simulink model "serial_send"  (R2018a)
settings: Solver=FixedStepAuto  StartTime=0.0  StopTime=1000000  FixedStep=0.01  RelTol=1e-3
undefined symbols (not defined in the file): serial
libraries: instrumentlib x2
settings Model: Creator=SIMONE  LastModifiedBy=SIMONE

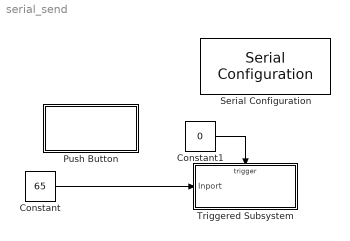
== system serial_send ==
  Constant : Constant  Value=65  OutDataTypeStr=uint8
  Constant1 : Constant  Value=0
  Push Button : Subsystem  DialogController=hmiCreateDDGDialog  IsWebBlock=on  mask(MWDashboardBlock){webBlockId=902a047b-b66d-44d2-ba72-a48565075944, webBlockType=pushbutton, ShowInLibBrwoser=on, ShowInitialText=on, HMISrcModelName=serial_send}
      mask prompts: webBlockId "WebBlock Id"; webBlockType "WebBlock Type"; HMISrcModelName "Source Model"
      mask help: SimulinkHMI:dialogs:PushButtonDialogDesc
      mask Help: helpview([docroot '/mapfiles/simulink.map'], 'hmi_push_button')
      mask Display:
      | model = bdroot(gcb);
      | if strcmp(get_param(model,'BlockDiagramType'), 'library')
      |     image([(matlabroot) '/toolbox/simulink/hmi/icons/PushButton.png']);
      | end
  Serial Configuration : instrumentlib/Serial Configuration  Priority=-200000  ComPortMenu=COM4  ComPort=COM4  ObjConstructor=serial('COM4');  BaudRate=115200  DataBits=8  Parity=none  StopBits=1  FlowControl=none  Timeout=10  ByteOrder=LittleEndian
  Triggered Subsystem : Subsystem  TreatAsAtomicUnit=on
  wires:
  Constant/1 -> Triggered Subsystem/1(Inport)
  Constant1/1 -> Triggered Subsystem/Trigger

== system serial_send/Push Button ==

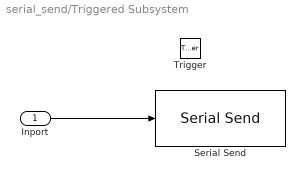
== system serial_send/Triggered Subsystem ==
  Inport : Inport
  Trigger : TriggerPort  VariantControl=Variant
  Serial Send : instrumentlib/Serial Send  ComPortMenu=COM4  ComPort=COM4  ObjConstructor=serial('COM4');  Terminator=<none>  EnableBlockingMode=on
  wires:
  Inport/1 -> Serial Send/1
